simulink model "Acce_Ctrl"  (R2017a)
settings: Solver=VariableStepAuto  StartTime=0.0  StopTime=12  RelTol=1e-3
settings Model: Creator=f26025  LastModifiedBy=f26025

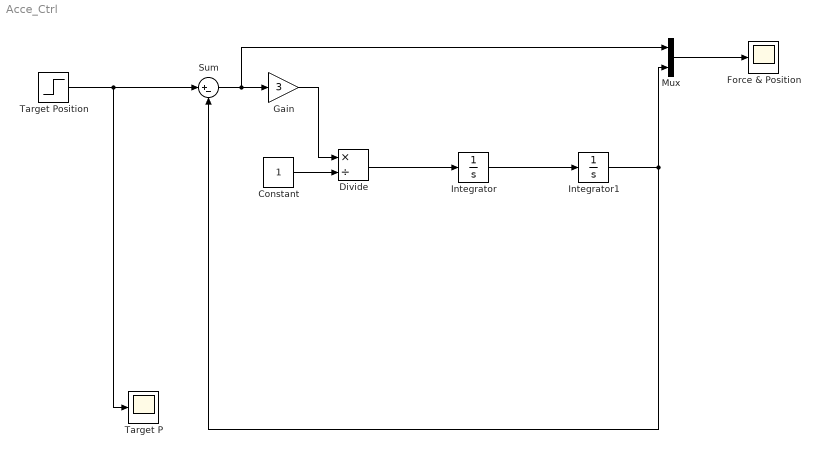
== system Acce_Ctrl ==
  Constant : Constant
  Divide : Product  Inputs=*/
  "Force & Position " : Scope
  Gain : Gain  Gain=3
  Integrator : Integrator
  Integrator1 : Integrator
  Mux : Mux  Inputs=2
  Sum : Sum  Inputs=|+-
  Target P : Scope
  Target Position : Step  SampleTime=0
  wires:
  Constant/1 -> Divide/2
  Integrator/1 -> Integrator1/1
  Integrator1/1 -> Sum/2, Mux/2
  Divide/1 -> Integrator/1
  Gain/1 -> Divide/1
  Target Position/1 -> Target P/1, Sum/1
  Sum/1 -> Mux/1, Gain/1
  Mux/1 -> "Force & Position "/1
